simulink model "vertical_control"  (Simulink 7.6)
settings: Solver=FixedStepDiscrete  StartTime=0.0  StopTime=Tfin  FixedStep=Ts  RelTol=1e-3
undefined symbols (not defined in the file or in its folder): airspeed_trim, DiscIntNeverNeededParam, elevators_max, elevators_min, elevators_trim, K_alt, K_vpath, mph2fps, pitch_trim, pitchrate_trim, vpath_trim
settings Model: Creator=borjafons  LastModifiedBy=frafonal
settings OptimizationCC: InlineParams=on  OptimizeModelRefInitCode=on  LifeSpan=1
settings DebuggingCC: FcnCallInpInsideContextMsg=Enable All
settings RTWCC: SystemTargetFile=ert.tlc  GenCodeOnly=on  TemplateMakefile=ert_default_tmf  Description=Embedded Coder  ProcessScript=ert_make_rtw_hook
settings CodeAppCC: IgnoreCustomStorageClasses=off
settings ERTTargetCC: MultiwordLength=2048  GenerateSampleERTMain=on  SupportNonFinite=off  SupportComplex=off  InlinedParameterPlacement=NonHierarchical  ERTCustomFileTemplate=example_file_process.tlc  ConvertIfToSwitch=off

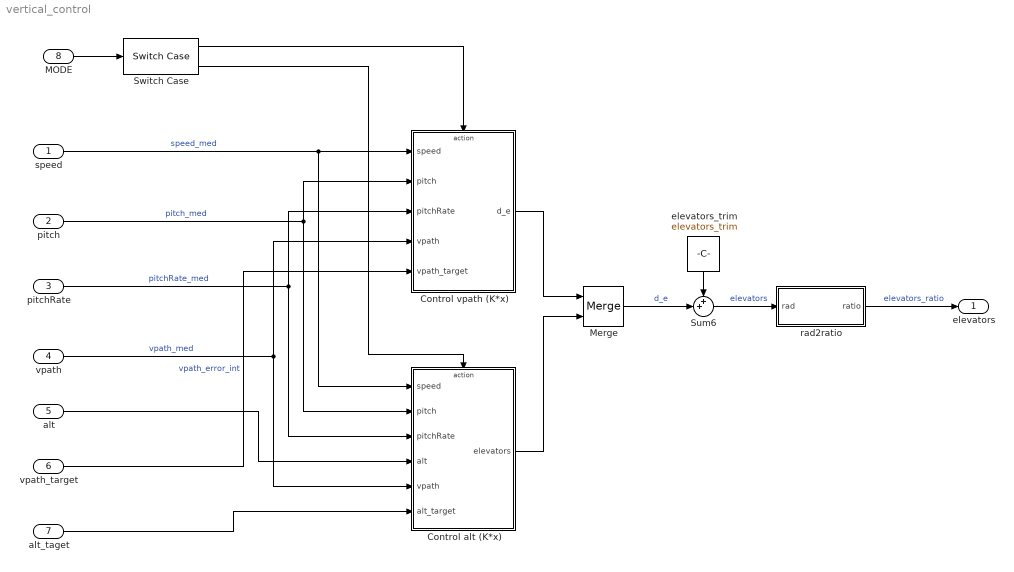
== system vertical_control ==
  speed : Inport  OutDataTypeStr=double
  pitch : Inport  Port=2  OutDataTypeStr=double
  pitchRate : Inport  Port=3  OutDataTypeStr=double
  vpath : Inport  Port=4  OutDataTypeStr=double
  alt : Inport  Port=5  OutDataTypeStr=double
  vpath_target : Inport  Port=6  OutDataTypeStr=double
  alt_taget : Inport  Port=7  OutDataTypeStr=double
  MODE : Inport  Port=8  OutDataTypeStr=double
  Control alt (K*x) : Subsystem  TreatAsAtomicUnit=on
  Control vpath (K*x) : Subsystem  TreatAsAtomicUnit=on
  Merge : Merge
  Sum6 : Sum  Inputs=++|
  Switch Case : SwitchCase  CaseConditions={VPATH_CONTROL, ALT_CONTROL}  ShowDefaultCase=off
  elevators_trim : Constant  Value=elevators_trim
  rad2ratio : Subsystem
  elevators : Outport
  wires:
  elevators_trim/1 -> Sum6/1
  Merge/1 -> Sum6/2  "d_e"
  rad2ratio/1(ratio) -> elevators/1  "elevators_ratio"
  Sum6/1 -> rad2ratio/1(rad)  "elevators"
  MODE/1 -> Switch Case/1
  Control vpath (K*x)/1(d_e) -> Merge/1
  Control alt (K*x)/1(elevators) -> Merge/2
  Switch Case/1 -> Control vpath (K*x)/Action
  Switch Case/2 -> Control alt (K*x)/Action
  speed/1 -> Control vpath (K*x)/1(speed), Control alt (K*x)/1(speed)  "speed_med"
  pitch/1 -> Control vpath (K*x)/2(pitch), Control alt (K*x)/2(pitch)  "pitch_med"
  pitchRate/1 -> Control vpath (K*x)/3(pitchRate), Control alt (K*x)/3(pitchRate)  "pitchRate_med"
  vpath/1 -> Control vpath (K*x)/4(vpath), Control alt (K*x)/5(vpath)  "vpath_med"
  alt/1 -> Control alt (K*x)/4(alt)
  vpath_target/1 -> Control vpath (K*x)/5(vpath_target)  "vpath_error_int"
  alt_taget/1 -> Control alt (K*x)/6(alt_target)

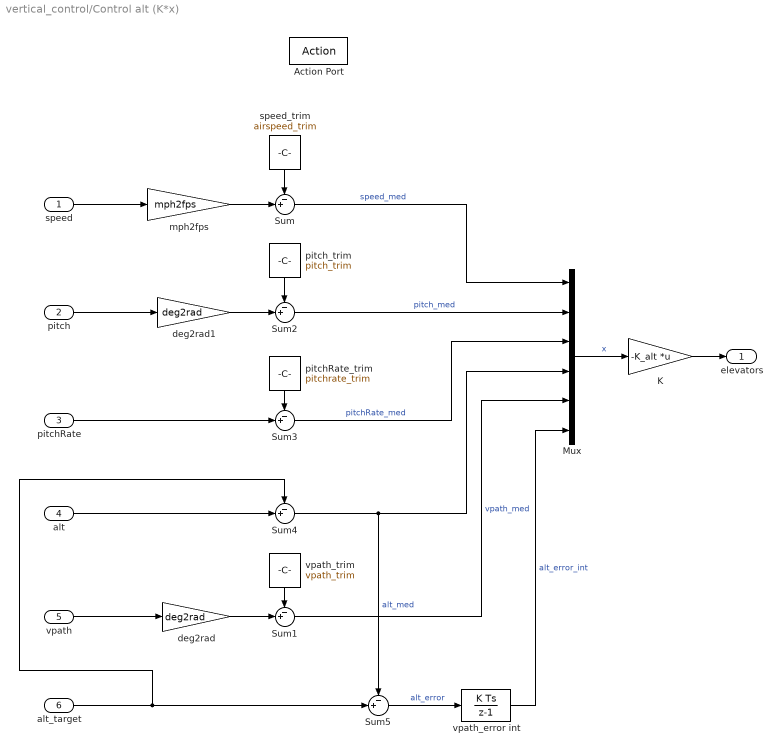
== system vertical_control/Control alt (K*x) ==
  speed : Inport  OutDataTypeStr=double
  pitch : Inport  Port=2  OutDataTypeStr=double
  pitchRate : Inport  Port=3  OutDataTypeStr=double
  alt : Inport  Port=4  OutDataTypeStr=double
  vpath : Inport  Port=5  OutDataTypeStr=double
  alt_target : Inport  Port=6  OutDataTypeStr=double
  Action Port : ActionPort  ActionType=case
  K : Gain  Gain=-K_alt  Multiplication=Matrix(K*u) (u vector)
  Mux : Mux  Inputs=6
  Sum{,1..5} (6 alike) : Sum  Inputs=-+|
  deg2rad : Gain  Gain=deg2rad
  deg2rad1 : Gain  Gain=deg2rad
  mph2fps : Gain  Gain=mph2fps  OutDataTypeStr=Inherit: Same as input
  pitchRate_trim : Constant  Value=pitchrate_trim
  pitch_trim : Constant  Value=pitch_trim
  speed_trim : Constant  Value=airspeed_trim
  vpath_error int : DiscreteIntegrator  SampleTime=-1  LimitOutput=on  UpperSaturationLimit=10  LowerSaturationLimit=-10  ICPrevOutput=DiscIntNeverNeededParam  ICPrevScaledInput=DiscIntNeverNeededParam
  vpath_trim : Constant  Value=vpath_trim
  elevators : Outport
  wires:
  speed/1 -> mph2fps/1
  vpath/1 -> deg2rad/1
  pitch/1 -> deg2rad1/1
  pitch_trim/1 -> Sum2/1
  vpath_trim/1 -> Sum1/1
  speed_trim/1 -> Sum/1
  deg2rad1/1 -> Sum2/2
  deg2rad/1 -> Sum1/2
  mph2fps/1 -> Sum/2
  pitchRate_trim/1 -> Sum3/1
  pitchRate/1 -> Sum3/2
  Sum/1 -> Mux/1  "speed_med"
  Sum2/1 -> Mux/2  "pitch_med"
  Sum3/1 -> Mux/3  "pitchRate_med"
  alt_target/1 -> Sum5/2, Sum4/1
  Sum5/1 -> vpath_error int/1  "alt_error"
  Mux/1 -> K/1  "x"
  K/1 -> elevators/1
  alt/1 -> Sum4/2
  Sum4/1 -> Mux/4, Sum5/1  "alt_med"
  Sum1/1 -> Mux/5  "vpath_med"
  vpath_error int/1 -> Mux/6  "alt_error_int"

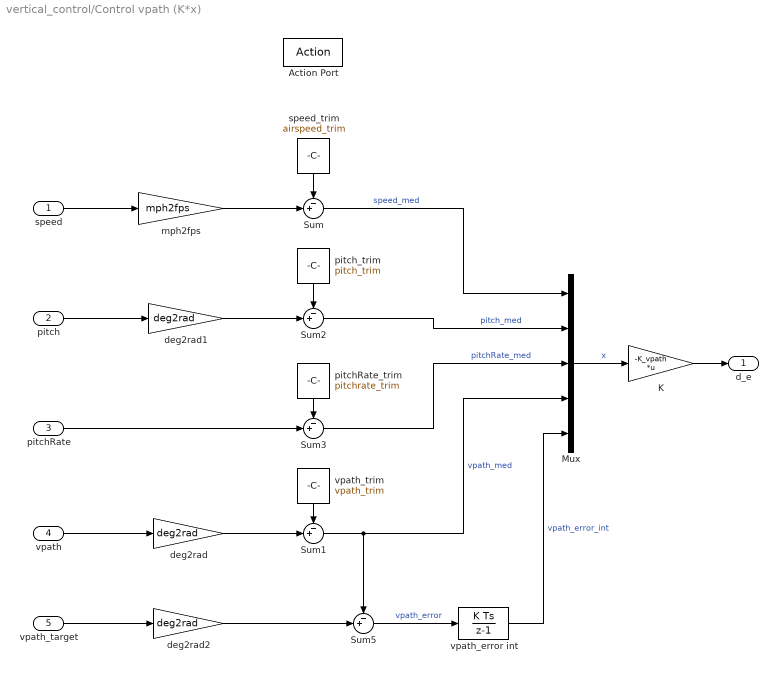
== system vertical_control/Control vpath (K*x) ==
  speed : Inport  OutDataTypeStr=double
  pitch : Inport  Port=2  OutDataTypeStr=double
  pitchRate : Inport  Port=3  OutDataTypeStr=double
  vpath : Inport  Port=4  OutDataTypeStr=double
  vpath_target : Inport  Port=5  OutDataTypeStr=double
  Action Port : ActionPort  ActionType=case
  K : Gain  Gain=-K_vpath  Multiplication=Matrix(K*u) (u vector)
  Mux : Mux  Inputs=5
  Sum{,1..3,5} (5 alike) : Sum  Inputs=-+|
  deg2rad : Gain  Gain=deg2rad
  deg2rad1 : Gain  Gain=deg2rad
  deg2rad2 : Gain  Gain=deg2rad
  mph2fps : Gain  Gain=mph2fps  OutDataTypeStr=Inherit: Same as input
  pitchRate_trim : Constant  Value=pitchrate_trim
  pitch_trim : Constant  Value=pitch_trim
  speed_trim : Constant  Value=airspeed_trim
  vpath_error int : DiscreteIntegrator  SampleTime=-1  LimitOutput=on  UpperSaturationLimit=10  LowerSaturationLimit=-10  ICPrevOutput=DiscIntNeverNeededParam  ICPrevScaledInput=DiscIntNeverNeededParam
  vpath_trim : Constant  Value=vpath_trim
  d_e : Outport
  wires:
  speed/1 -> mph2fps/1
  vpath/1 -> deg2rad/1
  pitch/1 -> deg2rad1/1
  pitch_trim/1 -> Sum2/1
  vpath_trim/1 -> Sum1/1
  speed_trim/1 -> Sum/1
  deg2rad1/1 -> Sum2/2
  deg2rad/1 -> Sum1/2
  mph2fps/1 -> Sum/2
  pitchRate_trim/1 -> Sum3/1
  pitchRate/1 -> Sum3/2
  Sum/1 -> Mux/1  "speed_med"
  Sum2/1 -> Mux/2  "pitch_med"
  Sum3/1 -> Mux/3  "pitchRate_med"
  Sum1/1 -> Mux/4, Sum5/1  "vpath_med"
  vpath_target/1 -> deg2rad2/1
  Sum5/1 -> vpath_error int/1  "vpath_error"
  Mux/1 -> K/1  "x"
  vpath_error int/1 -> Mux/5  "vpath_error_int"
  deg2rad2/1 -> Sum5/2
  K/1 -> d_e/1

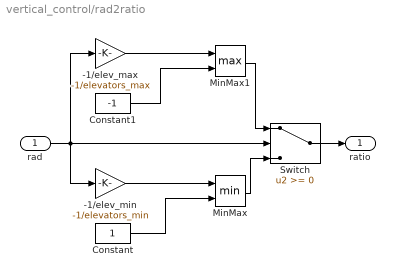
== system vertical_control/rad2ratio ==
  rad : Inport
  -1/elev_max : Gain  Gain=-1/elevators_max
  -1/elev_min : Gain  Gain=-1/elevators_min
  Constant : Constant
  Constant1 : Constant  Value=-1
  MinMax : MinMax  Inputs=2
  MinMax1 : MinMax  Function=max  Inputs=2
  Switch : Switch
  ratio : Outport
  wires:
  -1/elev_min/1 -> MinMax/1
  Constant/1 -> MinMax/2
  MinMax/1 -> Switch/3
  -1/elev_max/1 -> MinMax1/1
  Constant1/1 -> MinMax1/2
  MinMax1/1 -> Switch/1
  rad/1 -> Switch/2, -1/elev_min/1, -1/elev_max/1
  Switch/1 -> ratio/1
